simulink model "senior_project_final_3_9"  (Simulink 7.1)
settings: Solver=ode45  StartTime=0.0  StopTime=50e-6  RelTol=1e-3
libraries: xbsIndex_r4 x46, dspsrcs4 x1
settings Model: Creator=Danny  LastModifiedBy=Danny

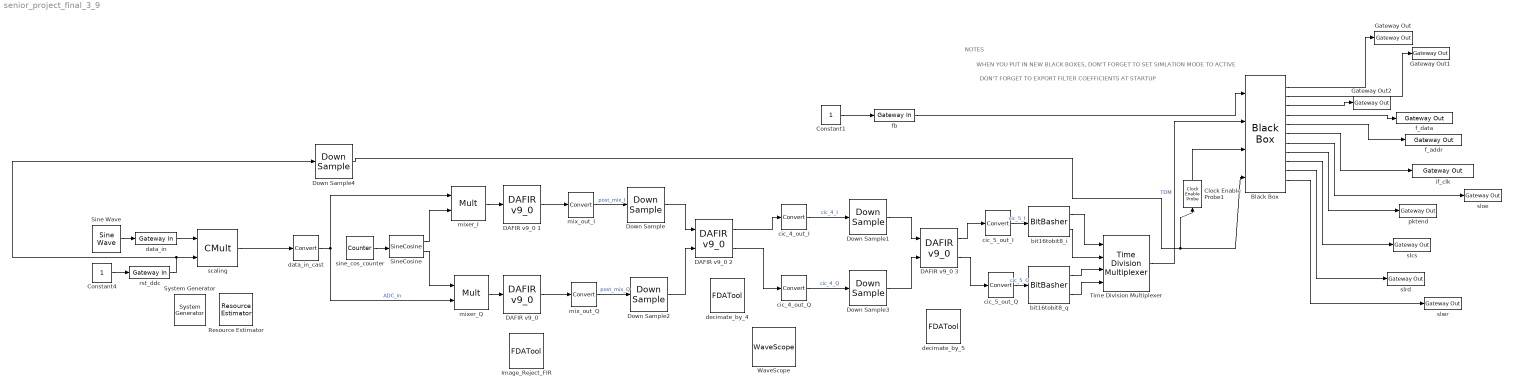
== system senior_project_final_3_9 ==
  note: WHEN YOU PUT IN NEW BLACK BOXES, DON'T FORGET TO SET SIMLATION MODE TO ACTIVE
  note: DON'T FORGET TO EXPORT FILTER COEFFICIENTS AT STARTUP
  note: NOTES
  " System Generator" : xbsIndex_r4/ System Generator  Tag=genX  SystemSampleTime=-1  xilinxfamily=spartan3e  part=xc3s500e  speed=-4  package=fg320  synthesis_tool=XST  clock_wrapper=Expose Clock Ports  directory=C:/Documents and Settings/Danny/Desktop/senior_project_5/netlist_senior_proj_final_3_9_2  testbench=on  simulink_period=1/(100e6)  sysclk_period=(1e9)/(100e6)  dcm_input_clock_period=100  incr_netlist=off  trim_vbits=Everywhere in SubSystem  dbl_ovrd=According to Block Masks  core_generation=According to Block Masks  run_coregen=off  deprecated_control=off  eval_field=0  block_type=sysgen
      settings: block_version=10.1.3
  Black Box : xbsIndex_r4/Black Box  init_code=usb_controller_final_2_config  sim_method=ISE Simulator  block_type=blackbox2
      settings: infoedit="Incorporates black box HDL and simulation model into a System Generator design.<P><P>You must supply a Black Box with certain information about the HDL component you would like to bring into System Generator. This information is provided through a Matlab function.<P><P>When \"Simulation mode\" is set to \"Inactive\", you will typically want to provide a separate simulation model by using a Simulation Multiplexer.<P>When \"Simulation mode\" is set to \"External co-simulator\", you must include a ModelSim block in the design."  xl_area=[16 18 0 29 0 0 0]  block_version=10.1.3
  Clock Enable Probe1 : xbsIndex_r4/Clock Enable Probe  Orientation=up  block_type=ceprobe
      settings: infoedit="Clock enable extractor.  Produces a Boolean output that mirrors the hardware clock enable associated with the input sample rate.<P><P>Hardware notes: in hardware this block costs nothing."  block_version=10.1.3
  Constant1 : Constant  OutDataType=sfix(16)  OutScaling=2^0
  Constant4 : Constant  OutDataType=sfix(16)  OutScaling=2^0
  "DAFIR v9_0 " : xbsIndex_r4/DAFIR v9_0   coef=|  structure=Inferred from Coefficients  coef_n_bits=16  coef_bin_pt=14  over_sample=1  reload=off  valids=off  rst=off  latency=14  num_channels=1  serial_input=off  polyphase_behavior="Single Rate:  sample in - sample out"  dbl_ovrd=off  explicit_period=off  period=1  use_isim=0  block_type=fir
      | [0.000686959913669627	0.00356456521897378	0.0109618965587764	0.0249428578248592	0.0456663374459672	0.0701211329273464	0.0923848852227348	0.105746394678378	0.105746394678378	0.0923848852227348	0.0701211329273464	0.0456663374459672	0.0249428578248592	0.0109618965587764	0.00356456521897378	0.000686959913669627
      | ]
      settings: infoedit="Hardware notes: Implemented using distributed arithmetic (DA).  The hardware over sampling rate determines the degree of parallelism.  A rate of one produces a fully parallel DA filter.  A rate of n (resp., n+1) for an n-bit input signal produces a fully serial implementation for a non-symmetric (resp., symmetric) impulse response.  Intermediate values produce implementations with intermediate levels of parallelism."  xl_use_area=on  xl_area=[803 1533 0 1124 0 0 0]  block_version=10.1.3
  DAFIR v9_0 1 : xbsIndex_r4/DAFIR v9_0   coef=|  structure=Inferred from Coefficients  coef_n_bits=16  coef_bin_pt=14  over_sample=1  reload=off  valids=off  rst=off  latency=14  num_channels=1  serial_input=off  polyphase_behavior="Single Rate:  sample in - sample out"  dbl_ovrd=off  explicit_period=off  period=1  use_isim=0  block_type=fir
      | [0.000686959913669627	0.00356456521897378	0.0109618965587764	0.0249428578248592	0.0456663374459672	0.0701211329273464	0.0923848852227348	0.105746394678378	0.105746394678378	0.0923848852227348	0.0701211329273464	0.0456663374459672	0.0249428578248592	0.0109618965587764	0.00356456521897378	0.000686959913669627
      | ]
      settings: infoedit="Hardware notes: Implemented using distributed arithmetic (DA).  The hardware over sampling rate determines the degree of parallelism.  A rate of one produces a fully parallel DA filter.  A rate of n (resp., n+1) for an n-bit input signal produces a fully serial implementation for a non-symmetric (resp., symmetric) impulse response.  Intermediate values produce implementations with intermediate levels of parallelism."  xl_use_area=on  xl_area=[803 1533 0 1124 0 0 0]  block_version=10.1.3
  DAFIR v9_0 2 : xbsIndex_r4/DAFIR v9_0   coef=|  structure=Inferred from Coefficients  coef_n_bits=16  coef_bin_pt=14  over_sample=1  reload=off  valids=off  rst=off  latency=13  num_channels=2  serial_input=off  polyphase_behavior="Single Rate:  sample in - sample out"  dbl_ovrd=off  explicit_period=off  period=1  use_isim=0  block_type=fir
      | [0.00347460557627437	0.0144082175652413	0.0368111171148552	0.0702919002348481	0.108007108573204	0.138258289953759	0.149875944396024	0.138258289953759	0.108007108573204	0.0702919002348481	0.0368111171148552	0.0144082175652413	0.00347460557627437
      | ]
      settings: infoedit="Hardware notes: Implemented using distributed arithmetic (DA).  The hardware over sampling rate determines the degree of parallelism.  A rate of one produces a fully parallel DA filter.  A rate of n (resp., n+1) for an n-bit input signal produces a fully serial implementation for a non-symmetric (resp., symmetric) impulse response.  Intermediate values produce implementations with intermediate levels of parallelism."  xl_area=[1171 2193 0 1819 0 0 0]  block_version=10.1.3
  DAFIR v9_0 3 : xbsIndex_r4/DAFIR v9_0   coef=|  structure=Inferred from Coefficients  coef_n_bits=16  coef_bin_pt=14  over_sample=1  reload=off  valids=off  rst=off  latency=13  num_channels=2  serial_input=off  polyphase_behavior="Single Rate:  sample in - sample out"  dbl_ovrd=off  explicit_period=off  period=1  use_isim=0  block_type=fir
      | [-0.0347987420721436	0	0.284550817173753	0.500000000000000	0.284550817173753	0	-0.0347987420721436
      | ]
      settings: infoedit="Hardware notes: Implemented using distributed arithmetic (DA).  The hardware over sampling rate determines the degree of parallelism.  A rate of one produces a fully parallel DA filter.  A rate of n (resp., n+1) for an n-bit input signal produces a fully serial implementation for a non-symmetric (resp., symmetric) impulse response.  Intermediate values produce implementations with intermediate levels of parallelism."  xl_area=[768 1313 0 859 0 0 0]  block_version=10.1.3
  Down Sample : xbsIndex_r4/Down Sample  sample_ratio=4  sample_phase="Last Value of Frame  (most efficient)"  en=off  latency=1  dbl_ovrd=off  block_type=dsamp
      settings: xl_area=[10 19 0 0 0 0 0]  block_version=10.1.3
  Down Sample1 : xbsIndex_r4/Down Sample  sample_ratio=5  sample_phase="Last Value of Frame  (most efficient)"  en=off  latency=1  dbl_ovrd=off  block_type=dsamp
      settings: xl_area=[10 19 0 0 0 0 0]  block_version=10.1.3
  Down Sample2 : xbsIndex_r4/Down Sample  sample_ratio=4  sample_phase="Last Value of Frame  (most efficient)"  en=off  latency=1  dbl_ovrd=off  block_type=dsamp
      settings: xl_area=[10 19 0 0 0 0 0]  block_version=10.1.3
  Down Sample3 : xbsIndex_r4/Down Sample  sample_ratio=5  sample_phase="Last Value of Frame  (most efficient)"  en=off  latency=1  dbl_ovrd=off  block_type=dsamp
      settings: xl_area=[10 19 0 0 0 0 0]  block_version=10.1.3
  Down Sample4 : xbsIndex_r4/Down Sample  sample_ratio=5  sample_phase="Last Value of Frame  (most efficient)"  en=off  latency=1  dbl_ovrd=off  block_type=dsamp
      settings: xl_area=[1 1 0 0 0 0 0]  block_version=10.1.3
  Gateway Out : xbsIndex_r4/Gateway Out  hdl_port=on  timing_constraint=None  locs_specified=off  LOCs={'P15'}  block_type=gatewayout
      settings: infoedit="Gateway out block.  Converts Xilinx fixed point inputs into ouputs of type Simulink integer, double, or fixed point.<P><P>Hardware notes:  In hardware these blocks become top level output ports or are discarded, depending on how they are configured."  block_version=10.1.3
  Gateway Out1 : xbsIndex_r4/Gateway Out  hdl_port=on  timing_constraint=None  locs_specified=off  LOCs={'F4'}  block_type=gatewayout
      settings: infoedit="Gateway out block.  Converts Xilinx fixed point inputs into ouputs of type Simulink integer, double, or fixed point.<P><P>Hardware notes:  In hardware these blocks become top level output ports or are discarded, depending on how they are configured."  block_version=10.1.3
  Gateway Out2 : xbsIndex_r4/Gateway Out  hdl_port=on  timing_constraint=None  locs_specified=off  LOCs={'R4'}  block_type=gatewayout
      settings: infoedit="Gateway out block.  Converts Xilinx fixed point inputs into ouputs of type Simulink integer, double, or fixed point.<P><P>Hardware notes:  In hardware these blocks become top level output ports or are discarded, depending on how they are configured."  block_version=10.1.3
  Image_Reject_FIR : xbsIndex_r4/FDATool  block_type=fdatool
      settings: infoedit=FDATool  block_version=10.1.3
  Resource Estimator : xbsIndex_r4/Resource Estimator  Tag=resEstTag  Slices=3939  FFs=7084  BRAMs=2  LUTs=5402  IOBs=37  EBMs=8  TBUFs=0  xl_use_estimator_area=off  est_options=Estimate  xl_estimator_area=[4347 7823 2 5897 130 8 0]  block_type=resource_estimator
      settings: AttributesFormatString=Resource\nEstimator  block_version=10.1.3
  Sine Wave : dspsrcs4/Sine Wave  Amplitude=20e-3  Frequency=20.1e6  Phase=0  SampleMode=Discrete  OutComplex=Real  CompMethod=Trigonometric fcn  TableSize=Speed  SampleTime=1/(100e6)  SamplesPerFrame=1  dataType=double  wordLen=16  udDataType=sfix(16)  fracBitsMode=Best precision  numFracBits=15  ResetState=Restart at time zero
  SineCosine : xbsIndex_r4/SineCosine  mode=Sine and Cosine  neg_sin=off  neg_cos=off  n_bits=19  sym_output=on  en=off  latency=1  dbl_ovrd=off  explicit_period=on  period=1/(100e6)  mem_type=Block RAM  pipeline=on  use_rpm=on  block_type=sincos
      settings: xl_area=[46 6 2 83 0 0 0]  block_version=10.1.3
  Time Division Multiplexer : xbsIndex_r4/Time Division Multiplexer  inputs=4  vin=off  dbl_ovrd=off  explicit_period=off  period=1  block_type=tdm
      settings: infoedit="Multiple inputs are sampled and  presented serially at the output."  xl_area=[5 3 0 36 0 0 0]  block_version=10.1.3
  WaveScope : xbsIndex_r4/WaveScope  block_type=wavescope
      settings: block_version=10.1.3
  bit16tobit8_i : xbsIndex_r4/BitBasher  bitexpr=|  display_expr=off  sr_1=1  arith_type1=Unsigned  bin_pt1=0  sr_2=2  arith_type2=Unsigned  bin_pt2=0  sr_3=3  arith_type3=Unsigned  bin_pt3=0  sr_4=4  arith_type4=Unsigned  bin_pt4=0  dbl_ovrd=off  block_type=bitbasher
      | <html><head><meta name="qrichtext" content="1" /><style type="text/css">
      | p, li { white-space: pre-wrap; }
      | </style></head><body style=" font-family:'MS Shell Dlg 2'; font-size:8.25pt; font-weight:400; font-style:normal;">
      | <p style=" margin-top:12px; margin-bottom:12px; margin-left:0px; margin-right:0px; -qt-block-indent:0; text-indent:0px; font-family:'MS Shell Dlg'; font-size:8pt;">b = {a[15:8]};<br />c = {a[7:0]};</p></body></html>
      settings: block_version=10.1.3
  bit16tobit8_q : xbsIndex_r4/BitBasher  bitexpr=|  display_expr=off  sr_1=1  arith_type1=Unsigned  bin_pt1=0  sr_2=2  arith_type2=Unsigned  bin_pt2=0  sr_3=3  arith_type3=Unsigned  bin_pt3=0  sr_4=4  arith_type4=Unsigned  bin_pt4=0  dbl_ovrd=off  block_type=bitbasher
      | <html><head><meta name="qrichtext" content="1" /><style type="text/css">
      | p, li { white-space: pre-wrap; }
      | </style></head><body style=" font-family:'MS Shell Dlg 2'; font-size:8.25pt; font-weight:400; font-style:normal;">
      | <p style=" margin-top:12px; margin-bottom:12px; margin-left:0px; margin-right:0px; -qt-block-indent:0; text-indent:0px; font-family:'MS Shell Dlg'; font-size:8pt;">b = {a[15:8]};<br />c = {a[7:0]};</p></body></html>
      settings: block_version=10.1.3
  cic_4_out_I : xbsIndex_r4/Convert  arith_type="Signed  (2's comp)"  n_bits=16  bin_pt=14  quantization="Round  (unbiased: +/- Inf)"  overflow=Wrap  latency=0  dbl_ovrd=off  pipeline=off  block_type=convert
      settings: xl_area=[16 0 0 25 0 0 0]  block_version=VER_STRING_GOES_HERE
  cic_4_out_Q : xbsIndex_r4/Convert  arith_type="Signed  (2's comp)"  n_bits=16  bin_pt=14  quantization="Round  (unbiased: +/- Inf)"  overflow=Wrap  latency=0  dbl_ovrd=off  pipeline=off  block_type=convert
      settings: xl_area=[16 0 0 25 0 0 0]  block_version=VER_STRING_GOES_HERE
  cic_5_out_I : xbsIndex_r4/Convert  arith_type="Signed  (2's comp)"  n_bits=16  bin_pt=14  quantization=Truncate  overflow=Wrap  latency=0  dbl_ovrd=off  pipeline=on  block_type=convert
      settings: xl_area=[0 0 0 0 0 0 0]  block_version=VER_STRING_GOES_HERE
  cic_5_out_Q : xbsIndex_r4/Convert  arith_type="Signed  (2's comp)"  n_bits=16  bin_pt=14  quantization=Truncate  overflow=Wrap  latency=0  dbl_ovrd=off  pipeline=on  block_type=convert
      settings: xl_area=[0 0 0 0 0 0 0]  block_version=VER_STRING_GOES_HERE
  data_in : xbsIndex_r4/Gateway In  arith_type="Signed  (2's comp)"  n_bits=16  bin_pt=14  quantization="Round  (unbiased: +/- Inf)"  overflow=Saturate  period=1/(100e6)  dbl_ovrd=off  timing_constraint=Data Rate  locs_specified=on  LOCs={'K12', 'L16', 'M14', 'M16', 'P17', 'R16', 'T18', 'U18', 'H15', 'F14', 'G16', 'J12', 'K14', 'K15', 'J15', 'J14'}  block_type=gatewayin
      settings: infoedit="Gateway in block.  Converts inputs of type Simulink integer, double and fixed point to  Xilinx fixed point type.<P><P>Hardware notes:  In hardware these blocks become top level input ports."  xl_area=[0 0 0 0 16 0 0]  block_version=10.1.3
  data_in_cast : xbsIndex_r4/Convert  arith_type="Signed  (2's comp)"  n_bits=19  bin_pt=17  quantization="Round  (unbiased: +/- Inf)"  overflow=Wrap  latency=0  dbl_ovrd=off  pipeline=off  block_type=convert
      settings: xl_area=[15 0 0 24 0 0 0]  block_version=VER_STRING_GOES_HERE
  decimate_by_4 : xbsIndex_r4/FDATool  block_type=fdatool
      settings: infoedit=FDATool  block_version=10.1.3
  decimate_by_5 : xbsIndex_r4/FDATool  block_type=fdatool
      settings: infoedit=FDATool  block_version=10.1.3
  f_addr : xbsIndex_r4/Gateway Out  hdl_port=on  timing_constraint="Data Rate;  Set 'FAST' Attribute"  locs_specified=on  LOCs={'V13', 'T14'}  block_type=gatewayout
      settings: infoedit="Gateway out block.  Converts Xilinx fixed point inputs into ouputs of type Simulink integer, double, or fixed point.<P><P>Hardware notes:  In hardware these blocks become top level output ports or are discarded, depending on how they are configured."  xl_area=[0 0 0 0 2 0 0]  block_version=10.1.3
  f_data : xbsIndex_r4/Gateway Out  hdl_port=on  timing_constraint="Data Rate;  Set 'FAST' Attribute"  locs_specified=on  LOCs={'R10', 'P10', 'R11', 'N11', 'T12', 'P13', 'R13', 'R14'}  block_type=gatewayout
      settings: infoedit="Gateway out block.  Converts Xilinx fixed point inputs into ouputs of type Simulink integer, double, or fixed point.<P><P>Hardware notes:  In hardware these blocks become top level output ports or are discarded, depending on how they are configured."  xl_area=[0 0 0 0 8 0 0]  block_version=10.1.3
  fb : xbsIndex_r4/Gateway In  arith_type=Boolean  n_bits=16  bin_pt=14  quantization="Round  (unbiased: +/- Inf)"  overflow=Saturate  period=1/(20e6)  dbl_ovrd=off  timing_constraint=Data Rate  locs_specified=on  LOCs={'U14'}  block_type=gatewayin
      settings: infoedit="Gateway in block.  Converts inputs of type Simulink integer, double and fixed point to  Xilinx fixed point type.<P><P>Hardware notes:  In hardware these blocks become top level input ports."  xl_area=[0 0 0 0 1 0 0]  block_version=10.1.3
  if_clk : xbsIndex_r4/Gateway Out  hdl_port=on  timing_constraint="Data Rate;  Set 'FAST' Attribute"  locs_specified=on  LOCs={'T15'}  block_type=gatewayout
      settings: infoedit="Gateway out block.  Converts Xilinx fixed point inputs into ouputs of type Simulink integer, double, or fixed point.<P><P>Hardware notes:  In hardware these blocks become top level output ports or are discarded, depending on how they are configured."  xl_area=[0 0 0 0 1 0 0]  block_version=10.1.3
  mix_out_I : xbsIndex_r4/Convert  arith_type="Signed  (2's comp)"  n_bits=16  bin_pt=14  quantization="Round  (unbiased: +/- Inf)"  overflow=Wrap  latency=0  dbl_ovrd=off  pipeline=off  block_type=convert
      settings: xl_area=[15 0 0 24 0 0 0]  block_version=VER_STRING_GOES_HERE
  mix_out_Q : xbsIndex_r4/Convert  arith_type="Signed  (2's comp)"  n_bits=16  bin_pt=14  quantization="Round  (unbiased: +/- Inf)"  overflow=Wrap  latency=0  dbl_ovrd=off  pipeline=off  block_type=convert
      settings: xl_area=[15 0 0 24 0 0 0]  block_version=VER_STRING_GOES_HERE
  mixer_I : xbsIndex_r4/Mult  precision=User Defined  arith_type="Signed  (2's comp)"  n_bits=16  bin_pt=14  quantization=Truncate  overflow=Wrap  en=off  latency=5  dbl_ovrd=off  use_behavioral_HDL=off  use_embedded=on  opt=Speed  optimum_pipeline=on  pipeline=on  use_rpm=on  placement_style=Triangular  block_type=mult
      settings: infoedit=Hardware notes: To use the internal pipeline stage of the dedicated multiplier you must select 'Pipeline for maximum performance'.  xl_area=[98 191 0 98 0 4 0]  block_version=10.1.3
  mixer_Q : xbsIndex_r4/Mult  precision=User Defined  arith_type="Signed  (2's comp)"  n_bits=16  bin_pt=14  quantization=Truncate  overflow=Wrap  en=off  latency=5  dbl_ovrd=off  use_behavioral_HDL=off  use_embedded=on  opt=Speed  optimum_pipeline=on  pipeline=on  use_rpm=on  placement_style=Triangular  block_type=mult
      settings: infoedit=Hardware notes: To use the internal pipeline stage of the dedicated multiplier you must select 'Pipeline for maximum performance'.  xl_area=[98 191 0 98 0 4 0]  block_version=10.1.3
  pktend : xbsIndex_r4/Gateway Out  hdl_port=on  timing_constraint=None  locs_specified=off  LOCs={'V12'}  block_type=gatewayout
      settings: infoedit="Gateway out block.  Converts Xilinx fixed point inputs into ouputs of type Simulink integer, double, or fixed point.<P><P>Hardware notes:  In hardware these blocks become top level output ports or are discarded, depending on how they are configured."  block_version=10.1.3
  rst_ddc : xbsIndex_r4/Gateway In  arith_type=Boolean  n_bits=16  bin_pt=14  quantization="Round  (unbiased: +/- Inf)"  overflow=Saturate  period=1/(100e6)  dbl_ovrd=off  timing_constraint=Data Rate  locs_specified=on  LOCs={'G18'}  block_type=gatewayin
      settings: infoedit="Gateway in block.  Converts inputs of type Simulink integer, double and fixed point to  Xilinx fixed point type.<P><P>Hardware notes:  In hardware these blocks become top level input ports."  xl_area=[0 0 0 0 1 0 0]  block_version=10.1.3
  scaling : xbsIndex_r4/CMult  const=1  const_n_bits=19  const_bin_pt=17  en=on  latency=1  precision=Full  arith_type="Signed  (2's comp)"  n_bits=16  bin_pt=14  quantization=Truncate  overflow=Wrap  dbl_ovrd=off  use_behavioral_HDL=off  mem_type=Distributed RAM  placement_style=Rectangular Shape  pipeline=off  use_rpm=off  block_type=cmult
      settings: xl_area=[8 16 0 0 0 0 0]  block_version=10.1.3
  sine_cos_counter : xbsIndex_r4/Counter  cnt_type=Free Running  cnt_to=Inf  operation=Up  start_count=0  cnt_by_val=25  arith_type="Signed  (2's comp)"  n_bits=10  bin_pt=3  load_pin=off  rst=off  en=off  explicit_period=on  period=1/(100e6)  dbl_ovrd=off  use_behavioral_HDL=off  use_rpm=on  implementation=Fabric  block_type=counter
      settings: xl_area=[5 10 0 10 0 0 0]
  slcs : xbsIndex_r4/Gateway Out  hdl_port=on  timing_constraint=None  locs_specified=off  LOCs={'T16'}  block_type=gatewayout
      settings: infoedit="Gateway out block.  Converts Xilinx fixed point inputs into ouputs of type Simulink integer, double, or fixed point.<P><P>Hardware notes:  In hardware these blocks become top level output ports or are discarded, depending on how they are configured."  block_version=10.1.3
  sloe : xbsIndex_r4/Gateway Out  hdl_port=on  timing_constraint=None  locs_specified=off  LOCs={'V15'}  block_type=gatewayout
      settings: infoedit="Gateway out block.  Converts Xilinx fixed point inputs into ouputs of type Simulink integer, double, or fixed point.<P><P>Hardware notes:  In hardware these blocks become top level output ports or are discarded, depending on how they are configured."  block_version=10.1.3
  slrd : xbsIndex_r4/Gateway Out  hdl_port=on  timing_constraint=None  locs_specified=off  LOCs={'N9'}  block_type=gatewayout
      settings: infoedit="Gateway out block.  Converts Xilinx fixed point inputs into ouputs of type Simulink integer, double, or fixed point.<P><P>Hardware notes:  In hardware these blocks become top level output ports or are discarded, depending on how they are configured."  block_version=10.1.3
  slwr : xbsIndex_r4/Gateway Out  hdl_port=on  timing_constraint=None  locs_specified=off  LOCs={'V9'}  block_type=gatewayout
      settings: infoedit="Gateway out block.  Converts Xilinx fixed point inputs into ouputs of type Simulink integer, double, or fixed point.<P><P>Hardware notes:  In hardware these blocks become top level output ports or are discarded, depending on how they are configured."  block_version=10.1.3
  wires:
  SineCosine/2 -> mixer_Q/1
  SineCosine/1 -> mixer_I/2
  sine_cos_counter/1 -> SineCosine/1
  mixer_I/1 -> DAFIR v9_0 1/1
  mixer_Q/1 -> "DAFIR v9_0 "/1
  data_in/1 -> scaling/1
  DAFIR v9_0 1/1 -> mix_out_I/1
  "DAFIR v9_0 "/1 -> mix_out_Q/1
  scaling/1 -> data_in_cast/1
  mix_out_I/1 -> Down Sample/1  "post_mix_I"
  mix_out_Q/1 -> Down Sample2/1  "post_mix_Q"
  data_in_cast/1 -> mixer_Q/2, mixer_I/1  "ADC_in"
  DAFIR v9_0 2/1 -> cic_4_out_I/1
  cic_4_out_I/1 -> Down Sample1/1  "cic_4_I"
  Down Sample/1 -> DAFIR v9_0 2/1
  Down Sample2/1 -> DAFIR v9_0 2/2
  DAFIR v9_0 2/2 -> cic_4_out_Q/1
  cic_4_out_Q/1 -> Down Sample3/1  "cic_4_Q"
  Down Sample1/1 -> DAFIR v9_0 3/1
  Down Sample3/1 -> DAFIR v9_0 3/2
  Sine Wave/1 -> data_in/1
  fb/1 -> Black Box/1
  Constant1/1 -> fb/1
  Constant4/1 -> rst_ddc/1
  rst_ddc/1 -> scaling/2, Down Sample4/1
  cic_5_out_I/1 -> bit16tobit8_i/1  "cic_5_I"
  bit16tobit8_i/1 -> Time Division Multiplexer/1
  bit16tobit8_i/2 -> Time Division Multiplexer/2
  cic_5_out_Q/1 -> bit16tobit8_q/1  "cic_5_Q"
  bit16tobit8_q/1 -> Time Division Multiplexer/3
  bit16tobit8_q/2 -> Time Division Multiplexer/4
  Down Sample4/1 -> Clock Enable Probe1/1, Black Box/4
  DAFIR v9_0 3/2 -> cic_5_out_Q/1
  DAFIR v9_0 3/1 -> cic_5_out_I/1
  Black Box/4 -> f_data/1
  Black Box/5 -> f_addr/1
  Black Box/6 -> if_clk/1
  Black Box/1 -> Gateway Out/1
  Black Box/2 -> Gateway Out1/1
  Black Box/3 -> Gateway Out2/1
  Black Box/7 -> sloe/1
  Black Box/8 -> pktend/1
  Black Box/9 -> slcs/1
  Black Box/10 -> slrd/1
  Black Box/11 -> slwr/1
  Time Division Multiplexer/1 -> Black Box/2  "TDM"
  Clock Enable Probe1/1 -> Black Box/3
